simulink model "simulinkCS"  (Simulink 7.4)
settings: Solver=ode45  StartTime=0.0  StopTime=10.0  RelTol=1e-3
(part 2 of 2)

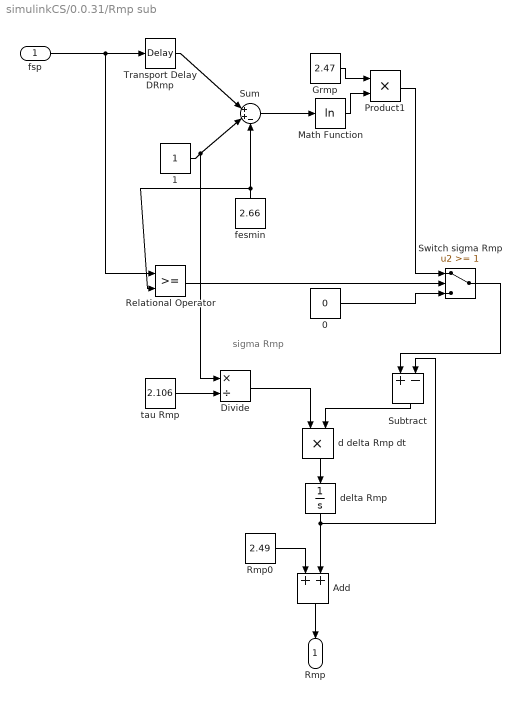
== system simulinkCS/0.0.31/Rmp sub ==
  note: sigma Rmp
  fsp : Inport  OutDataType=sfix(16)  OutScaling=2^0
  0 : Constant  Value=0  OutDataType=sfix(16)  OutScaling=2^0
  1 : Constant  OutDataType=sfix(16)  OutScaling=2^0
  Add : Sum  OutDataType=sfix(16)  OutScaling=2^-10
  Divide : Product  Inputs=*/  OutDataType=sfix(16)  OutScaling=2^-10
  Grmp : Constant  Value=2.47  OutDataType=sfix(16)  OutScaling=2^0
  Math Function : Math  Operator=log  OutDataType=sfix(16)  OutScaling=2^0  SaturateOnIntegerOverflow=on
  Product1 : Product  OutDataType=sfix(16)  OutScaling=2^0  RndMeth=Zero
  Relational Operator : RelationalOperator  LogicOutDataTypeMode=boolean  OutDataTypeStr=boolean
  Rmp0 : Constant  Value=2.49  OutDataType=sfix(16)  OutScaling=2^0
  Subtract : Sum  Inputs=+-  OutDataType=sfix(16)  OutScaling=2^-10
  Sum : Sum  Inputs=|++-  OutDataType=sfix(16)  OutScaling=2^0
  Switch sigma Rmp : Switch  Threshold=1
  Transport Delay DRmp : TransportDelay  DelayTime=2
  "d delta Rmp dt  " : Product  OutDataType=sfix(16)  OutScaling=2^0  RndMeth=Zero
  delta Rmp : Integrator
  fesmin : Constant  Value=2.66  OutDataType=sfix(16)  OutScaling=2^0
  tau Rmp : Constant  Value=2.106  OutDataType=sfix(16)  OutScaling=2^0
  Rmp : Outport  OutDataType=sfix(16)  OutScaling=2^0
  wires:
  fsp/1 -> Transport Delay DRmp/1, Relational Operator/1
  Grmp/1 -> Product1/1
  1/1 -> Sum/2, Divide/1
  fesmin/1 -> Sum/3, Relational Operator/2
  Transport Delay DRmp/1 -> Sum/1
  Sum/1 -> Math Function/1
  Math Function/1 -> Product1/2
  Product1/1 -> Switch sigma Rmp/1
  Relational Operator/1 -> Switch sigma Rmp/2
  0/1 -> Switch sigma Rmp/3
  Switch sigma Rmp/1 -> Subtract/1
  tau Rmp/1 -> Divide/2
  delta Rmp/1 -> Subtract/2, Add/2
  Subtract/1 -> "d delta Rmp dt  "/2
  Divide/1 -> "d delta Rmp dt  "/1
  "d delta Rmp dt  "/1 -> delta Rmp/1
  Rmp0/1 -> Add/1
  Add/1 -> Rmp/1

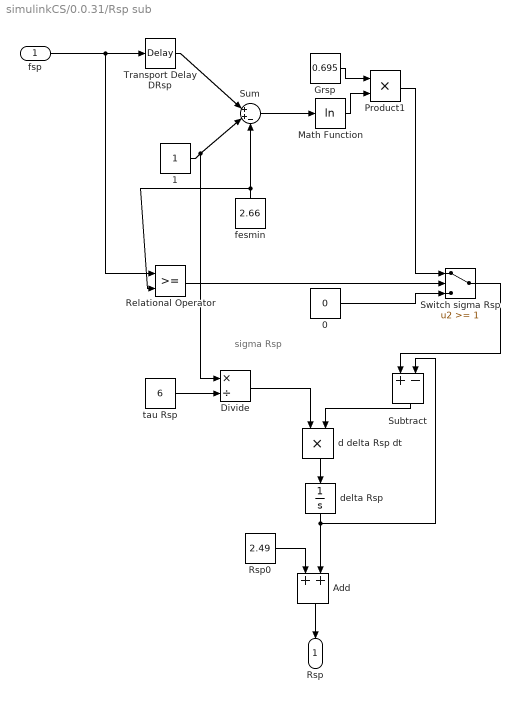
== system simulinkCS/0.0.31/Rsp sub ==
  note: sigma Rsp
  fsp : Inport  OutDataType=sfix(16)  OutScaling=2^0
  0 : Constant  Value=0  OutDataType=sfix(16)  OutScaling=2^0
  1 : Constant  OutDataType=sfix(16)  OutScaling=2^0
  Add : Sum  OutDataType=sfix(16)  OutScaling=2^-10
  Divide : Product  Inputs=*/  OutDataType=sfix(16)  OutScaling=2^-10
  Grsp : Constant  Value=0.695  OutDataType=sfix(16)  OutScaling=2^0
  Math Function : Math  Operator=log  OutDataType=sfix(16)  OutScaling=2^0  SaturateOnIntegerOverflow=on
  Product1 : Product  OutDataType=sfix(16)  OutScaling=2^0  RndMeth=Zero
  Relational Operator : RelationalOperator  LogicOutDataTypeMode=boolean  OutDataTypeStr=boolean
  Rsp0 : Constant  Value=2.49  OutDataType=sfix(16)  OutScaling=2^0
  Subtract : Sum  Inputs=+-  OutDataType=sfix(16)  OutScaling=2^-10
  Sum : Sum  Inputs=|++-  OutDataType=sfix(16)  OutScaling=2^0
  Switch sigma Rsp : Switch  Threshold=1
  Transport Delay DRsp : TransportDelay  DelayTime=2
  "d delta Rsp dt  " : Product  OutDataType=sfix(16)  OutScaling=2^0  RndMeth=Zero
  delta Rsp : Integrator
  fesmin : Constant  Value=2.66  OutDataType=sfix(16)  OutScaling=2^0
  tau Rsp : Constant  Value=6  OutDataType=sfix(16)  OutScaling=2^0
  Rsp : Outport  OutDataType=sfix(16)  OutScaling=2^0
  wires:
  fsp/1 -> Transport Delay DRsp/1, Relational Operator/1
  Grsp/1 -> Product1/1
  1/1 -> Sum/2, Divide/1
  fesmin/1 -> Sum/3, Relational Operator/2
  Transport Delay DRsp/1 -> Sum/1
  Sum/1 -> Math Function/1
  Math Function/1 -> Product1/2
  Product1/1 -> Switch sigma Rsp/1
  Relational Operator/1 -> Switch sigma Rsp/2
  0/1 -> Switch sigma Rsp/3
  Switch sigma Rsp/1 -> Subtract/1
  tau Rsp/1 -> Divide/2
  delta Rsp/1 -> Subtract/2, Add/2
  Subtract/1 -> "d delta Rsp dt  "/2
  Divide/1 -> "d delta Rsp dt  "/1
  "d delta Rsp dt  "/1 -> delta Rsp/1
  Rsp0/1 -> Add/1
  Add/1 -> Rsp/1

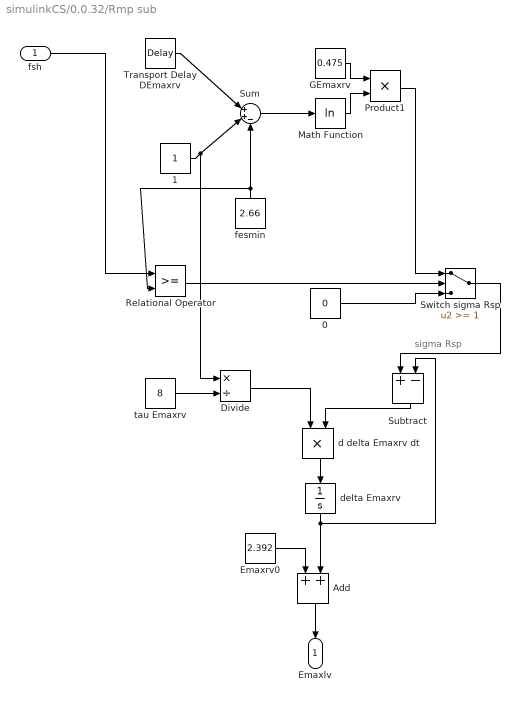
== system simulinkCS/0.0.32/Rmp sub ==
  note: sigma Rsp
  fsh : Inport  OutDataType=sfix(16)  OutScaling=2^0
  0 : Constant  Value=0  OutDataType=sfix(16)  OutScaling=2^0
  1 : Constant  OutDataType=sfix(16)  OutScaling=2^0
  Add : Sum  OutDataType=sfix(16)  OutScaling=2^-10
  Divide : Product  Inputs=*/  OutDataType=sfix(16)  OutScaling=2^-10
  Emaxrv0 : Constant  Value=2.392  OutDataType=sfix(16)  OutScaling=2^0
  GEmaxrv : Constant  Value=0.475  OutDataType=sfix(16)  OutScaling=2^0
  Math Function : Math  Operator=log  OutDataType=sfix(16)  OutScaling=2^0  SaturateOnIntegerOverflow=on
  Product1 : Product  OutDataType=sfix(16)  OutScaling=2^0  RndMeth=Zero
  Relational Operator : RelationalOperator  LogicOutDataTypeMode=boolean  OutDataTypeStr=boolean
  Subtract : Sum  Inputs=+-  OutDataType=sfix(16)  OutScaling=2^-10
  Sum : Sum  Inputs=|++-  OutDataType=sfix(16)  OutScaling=2^0
  Switch sigma Rsp : Switch  Threshold=1
  Transport Delay DEmaxrv : TransportDelay  DelayTime=2
  "d delta Emaxrv dt  " : Product  OutDataType=sfix(16)  OutScaling=2^0  RndMeth=Zero
  delta Emaxrv : Integrator
  fesmin : Constant  Value=2.66  OutDataType=sfix(16)  OutScaling=2^0
  tau Emaxrv : Constant  Value=8  OutDataType=sfix(16)  OutScaling=2^0
  Emaxlv : Outport  OutDataType=sfix(16)  OutScaling=2^0
  wires:
  fsh/1 -> Relational Operator/1
  GEmaxrv/1 -> Product1/1
  1/1 -> Sum/2, Divide/1
  fesmin/1 -> Sum/3, Relational Operator/2
  Transport Delay DEmaxrv/1 -> Sum/1
  Sum/1 -> Math Function/1
  Math Function/1 -> Product1/2
  Product1/1 -> Switch sigma Rsp/1
  Relational Operator/1 -> Switch sigma Rsp/2
  0/1 -> Switch sigma Rsp/3
  Switch sigma Rsp/1 -> Subtract/1
  tau Emaxrv/1 -> Divide/2
  delta Emaxrv/1 -> Subtract/2, Add/2
  Subtract/1 -> "d delta Emaxrv dt  "/2
  Divide/1 -> "d delta Emaxrv dt  "/1
  "d delta Emaxrv dt  "/1 -> delta Emaxrv/1
  Emaxrv0/1 -> Add/1
  Add/1 -> Emaxlv/1

== system simulinkCS/0.0.32/Rsp sub ==
  note: sigma Rsp
  fsh : Inport  OutDataType=sfix(16)  OutScaling=2^0
  0 : Constant  Value=0  OutDataType=sfix(16)  OutScaling=2^0
  1 : Constant  OutDataType=sfix(16)  OutScaling=2^0
  Add : Sum  OutDataType=sfix(16)  OutScaling=2^-10
  Divide : Product  Inputs=*/  OutDataType=sfix(16)  OutScaling=2^-10
  Emaxrv0 : Constant  Value=1.412  OutDataType=sfix(16)  OutScaling=2^0
  GEmaxrv : Constant  Value=0.282  OutDataType=sfix(16)  OutScaling=2^0
  Math Function : Math  Operator=log  OutDataType=sfix(16)  OutScaling=2^0  SaturateOnIntegerOverflow=on
  Product1 : Product  OutDataType=sfix(16)  OutScaling=2^0  RndMeth=Zero
  Relational Operator : RelationalOperator  LogicOutDataTypeMode=boolean  OutDataTypeStr=boolean
  Subtract : Sum  Inputs=+-  OutDataType=sfix(16)  OutScaling=2^-10
  Sum : Sum  Inputs=|++-  OutDataType=sfix(16)  OutScaling=2^0
  Switch sigma Rsp : Switch  Threshold=1
  Transport Delay DEmaxrv : TransportDelay  DelayTime=2
  "d delta Emaxrv dt  " : Product  OutDataType=sfix(16)  OutScaling=2^0  RndMeth=Zero
  delta Emaxrv : Integrator
  fesmin : Constant  Value=2.66  OutDataType=sfix(16)  OutScaling=2^0
  tau Emaxrv : Constant  Value=8  OutDataType=sfix(16)  OutScaling=2^0
  Emaxrv : Outport  OutDataType=sfix(16)  OutScaling=2^0
  wires:
  fsh/1 -> Transport Delay DEmaxrv/1, Relational Operator/1
  GEmaxrv/1 -> Product1/1
  1/1 -> Sum/2, Divide/1
  fesmin/1 -> Sum/3, Relational Operator/2
  Transport Delay DEmaxrv/1 -> Sum/1
  Sum/1 -> Math Function/1
  Math Function/1 -> Product1/2
  Product1/1 -> Switch sigma Rsp/1
  Relational Operator/1 -> Switch sigma Rsp/2
  0/1 -> Switch sigma Rsp/3
  Switch sigma Rsp/1 -> Subtract/1
  tau Emaxrv/1 -> Divide/2
  delta Emaxrv/1 -> Subtract/2, Add/2
  Subtract/1 -> "d delta Emaxrv dt  "/2
  Divide/1 -> "d delta Emaxrv dt  "/1
  "d delta Emaxrv dt  "/1 -> delta Emaxrv/1
  Emaxrv0/1 -> Add/1
  Add/1 -> Emaxrv/1

== system simulinkCS/0.0.34/Vumv sub ==
  note: sigma Vumv
  fsp : Inport  OutDataType=sfix(16)  OutScaling=2^0
  0 : Constant  Value=0  OutDataType=sfix(16)  OutScaling=2^0
  1 : Constant  OutDataType=sfix(16)  OutScaling=2^0
  Add : Sum  OutDataType=sfix(16)  OutScaling=2^-10
  Divide : Product  Inputs=*/  OutDataType=sfix(16)  OutScaling=2^-10
  GVumv : Constant  Value=-58.29  OutDataType=sfix(16)  OutScaling=2^0
  Math Function : Math  Operator=log  OutDataType=sfix(16)  OutScaling=2^0  SaturateOnIntegerOverflow=on
  Product1 : Product  OutDataType=sfix(16)  OutScaling=2^0  RndMeth=Zero
  Relational Operator : RelationalOperator  LogicOutDataTypeMode=boolean  OutDataTypeStr=boolean
  Subtract : Sum  Inputs=+-  OutDataType=sfix(16)  OutScaling=2^-10
  Sum : Sum  Inputs=|++-  OutDataType=sfix(16)  OutScaling=2^0
  Switch sigma Rsp : Switch  Threshold=1
  Transport Delay DVumv : TransportDelay  DelayTime=5
  Vumv0 : Constant  Value=503.26  OutDataType=sfix(16)  OutScaling=2^0
  "d delta Vumv dt  " : Product  OutDataType=sfix(16)  OutScaling=2^0  RndMeth=Zero
  delta Vumv : Integrator
  fesmin : Constant  Value=2.66  OutDataType=sfix(16)  OutScaling=2^0
  tau Rsp : Constant  Value=20  OutDataType=sfix(16)  OutScaling=2^0
  Vumv : Outport  OutDataType=sfix(16)  OutScaling=2^0
  wires:
  fsp/1 -> Transport Delay DVumv/1, Relational Operator/1
  GVumv/1 -> Product1/1
  1/1 -> Sum/2, Divide/1
  fesmin/1 -> Sum/3, Relational Operator/2
  Transport Delay DVumv/1 -> Sum/1
  Sum/1 -> Math Function/1
  Math Function/1 -> Product1/2
  Product1/1 -> Switch sigma Rsp/1
  Relational Operator/1 -> Switch sigma Rsp/2
  0/1 -> Switch sigma Rsp/3
  Switch sigma Rsp/1 -> Subtract/1
  tau Rsp/1 -> Divide/2
  delta Vumv/1 -> Subtract/2, Add/2
  Subtract/1 -> "d delta Vumv dt  "/2
  Divide/1 -> "d delta Vumv dt  "/1
  "d delta Vumv dt  "/1 -> delta Vumv/1
  Vumv0/1 -> Add/1
  Add/1 -> Vumv/1

== system simulinkCS/0.0.34/Vumv sub1 ==
  note: sigma Vumv
  fsp : Inport  OutDataType=sfix(16)  OutScaling=2^0
  0 : Constant  Value=0  OutDataType=sfix(16)  OutScaling=2^0
  1 : Constant  OutDataType=sfix(16)  OutScaling=2^0
  Add : Sum  OutDataType=sfix(16)  OutScaling=2^-10
  Divide : Product  Inputs=*/  OutDataType=sfix(16)  OutScaling=2^-10
  GVumv : Constant  Value=-74.21  OutDataType=sfix(16)  OutScaling=2^0
  Math Function : Math  Operator=log  OutDataType=sfix(16)  OutScaling=2^0  SaturateOnIntegerOverflow=on
  Product1 : Product  OutDataType=sfix(16)  OutScaling=2^0  RndMeth=Zero
  Relational Operator : RelationalOperator  LogicOutDataTypeMode=boolean  OutDataTypeStr=boolean
  Subtract : Sum  Inputs=+-  OutDataType=sfix(16)  OutScaling=2^-10
  Sum : Sum  Inputs=|++-  OutDataType=sfix(16)  OutScaling=2^0
  Switch sigma Rsp : Switch  Threshold=1
  Transport Delay DVumv : TransportDelay  DelayTime=5
  Vumv0 : Constant  Value=640.73  OutDataType=sfix(16)  OutScaling=2^0
  "d delta Vumv dt  " : Product  OutDataType=sfix(16)  OutScaling=2^0  RndMeth=Zero
  delta Vumv : Integrator
  fesmin : Constant  Value=2.66  OutDataType=sfix(16)  OutScaling=2^0
  tau Rsp : Constant  Value=20  OutDataType=sfix(16)  OutScaling=2^0
  Vusv : Outport  OutDataType=sfix(16)  OutScaling=2^0
  wires:
  fsp/1 -> Transport Delay DVumv/1, Relational Operator/1
  GVumv/1 -> Product1/1
  1/1 -> Sum/2, Divide/1
  fesmin/1 -> Sum/3, Relational Operator/2
  Transport Delay DVumv/1 -> Sum/1
  Sum/1 -> Math Function/1
  Math Function/1 -> Product1/2
  Product1/1 -> Switch sigma Rsp/1
  Relational Operator/1 -> Switch sigma Rsp/2
  0/1 -> Switch sigma Rsp/3
  Switch sigma Rsp/1 -> Subtract/1
  tau Rsp/1 -> Divide/2
  delta Vumv/1 -> Subtract/2, Add/2
  Subtract/1 -> "d delta Vumv dt  "/2
  Divide/1 -> "d delta Vumv dt  "/1
  "d delta Vumv dt  "/1 -> delta Vumv/1
  Vumv0/1 -> Add/1
  Add/1 -> Vusv/1

== system simulinkCS/0.0.34/Vumv sub2 ==
  note: sigma Vumv
  fsp : Inport  OutDataType=sfix(16)  OutScaling=2^0
  0 : Constant  Value=0  OutDataType=sfix(16)  OutScaling=2^0
  1 : Constant  OutDataType=sfix(16)  OutScaling=2^0
  Add : Sum  OutDataType=sfix(16)  OutScaling=2^-10
  Divide : Product  Inputs=*/  OutDataType=sfix(16)  OutScaling=2^-10
  GVumv : Constant  Value=-265.4  OutDataType=sfix(16)  OutScaling=2^0
  Math Function : Math  Operator=log  OutDataType=sfix(16)  OutScaling=2^0  SaturateOnIntegerOverflow=on
  Product1 : Product  OutDataType=sfix(16)  OutScaling=2^0  RndMeth=Zero
  Relational Operator : RelationalOperator  LogicOutDataTypeMode=boolean  OutDataTypeStr=boolean
  Subtract : Sum  Inputs=+-  OutDataType=sfix(16)  OutScaling=2^-10
  Sum : Sum  Inputs=|++-  OutDataType=sfix(16)  OutScaling=2^0
  Switch sigma Rsp : Switch  Threshold=1
  Transport Delay DVumv : TransportDelay  DelayTime=2
  Vumv0 : Constant  Value=1435.4  OutDataType=sfix(16)  OutScaling=2^0
  "d delta Vumv dt  " : Product  OutDataType=sfix(16)  OutScaling=2^0  RndMeth=Zero
  delta Vumv : Integrator
  fesmin : Constant  Value=2.66  OutDataType=sfix(16)  OutScaling=2^0
  tau Rsp : Constant  Value=20  OutDataType=sfix(16)  OutScaling=2^0
  Vuev : Outport  OutDataType=sfix(16)  OutScaling=2^0
  wires:
  fsp/1 -> Transport Delay DVumv/1, Relational Operator/1
  GVumv/1 -> Product1/1
  1/1 -> Sum/2, Divide/1
  fesmin/1 -> Sum/3, Relational Operator/2
  Transport Delay DVumv/1 -> Sum/1
  Sum/1 -> Math Function/1
  Math Function/1 -> Product1/2
  Product1/1 -> Switch sigma Rsp/1
  Relational Operator/1 -> Switch sigma Rsp/2
  0/1 -> Switch sigma Rsp/3
  Switch sigma Rsp/1 -> Subtract/1
  tau Rsp/1 -> Divide/2
  delta Vumv/1 -> Subtract/2, Add/2
  Subtract/1 -> "d delta Vumv dt  "/2
  Divide/1 -> "d delta Vumv dt  "/1
  "d delta Vumv dt  "/1 -> delta Vumv/1
  Vumv0/1 -> Add/1
  Add/1 -> Vuev/1

== system simulinkCS/A1.19 from michel/beta(H) ==
  H : Inport  OutDataType=sfix(16)  OutScaling=2^0
  alpha : Inport  Port=2  OutDataType=sfix(16)  OutScaling=2^0
  n : Inport  Port=3  OutDataType=sfix(16)  OutScaling=2^0
  m : Inport  Port=4  OutDataType=sfix(16)  OutScaling=2^0
  Add : Sum  OutDataType=sfix(16)  OutScaling=2^-10
  Add1 : Sum  Inputs=+-  OutDataType=sfix(16)  OutScaling=2^-10
  Divide : Product  Inputs=**/  OutDataType=sfix(16)  OutScaling=2^-10
  Product : Product  OutDataType=sfix(16)  OutScaling=2^0  RndMeth=Zero
  t p(H) : Fcn  Expr=0.1859+(1/(u^9.9+1))*(0.2799-0.1859)
  Out1 : Outport  OutDataType=sfix(16)  OutScaling=2^0
  wires:
  n/1 -> Add/1, Divide/3
  m/1 -> Add/2, Divide/2
  Add/1 -> Product/2
  t p(H)/1 -> Product/1
  H/1 -> t p(H)/1
  Product/1 -> Add1/1
  alpha/1 -> Divide/1
  Divide/1 -> Add1/2
  Add1/1 -> Out1/1

== matlab function A1.19 from michel/Embedded MATLAB Function ==
  data: t input double; y output double; Hmin input double
function y = fcn(t,Hmin)
% This block supports an embeddable subset of the MATLAB language.
% See the help menu for details. 

y = mod(t,60/Hmin);
